simulink model "PID_Regler"  (R2019a)
settings: Solver=VariableStepAuto  StartTime=0.0  StopTime=10.0  RelTol=1e-3
values from neighbouring files (symbols this model uses):
  b = 0.1    [inv_pend.m]
  g = 9.8    [inv_pend.m]
  I = 0.006    [inv_pend.m]
  l = 0.3    [inv_pend.m]
  m = 0.5    [inv_pend.m]
  M = 0.5    [inv_pend.m]
libraries: simulink x1
settings Model: Creator=Naveen  LastModifiedBy=Naveen

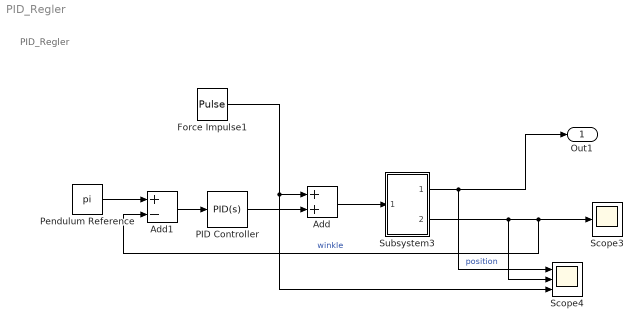
== system PID_Regler ==
  note: PID_Regler
  Add : Sum
  Add1 : Sum  Inputs=+-
  Force Impulse1 : DiscretePulseGenerator  PulseType=Time based  Amplitude=10  Period=100  PulseWidth=0.01  PhaseDelay=3
  PID Controller : simulink/Continuous/PID Controller  Controller=PID  Form=Parallel  TimeDomain=Continuous-time  SampleTime=-1  IntegratorMethod=Forward Euler  FilterMethod=Forward Euler  ControllerParametersSource=internal  P=100  I=1  D=20  UseFilter=on  N=100  TunerSelectOption=Transfer Function Based (PID Tuner App)  InitialConditionSource=internal  InitialConditionForIntegrator=0  InitialConditionForFilter=0  DifferentiatorICPrevScaledInput=0  ExternalReset=none  TrackingMode=off  Kt=1  LimitOutput=off  UpperSaturationLimit=inf  LowerSaturationLimit=-inf  LinearizeAsGain=on  AntiWindupMode=none  Kb=1  POutMin=[]  POutMax=[]  IOutMin=[]  IOutMax=[]  DOutMin=[]  DOutMax=[]  NOutMin=[]  NOutMax=[]  SumOutMin=[]  SumOutMax=[]  SaturationOutMin=[]  SaturationOutMax=[]  PParamMin=[]  PParamMax=[]  IParamMin=[]  IParamMax=[]  DParamMin=[]  DParamMax=[]  NParamMin=[]  NParamMax=[]  KbParamMin=[]  KbParamMax=[]  KtParamMin=[]  KtParamMax=[]  KbOutMin=[]  KbOutMax=[]  KtOutMin=[]  KtOutMax=[]  IntegratorOutMin=[]  IntegratorOutMax=[]  FilterOutMin=[]  FilterOutMax=[]  SumI1OutMin=[]  SumI1OutMax=[]  SumI2OutMin=[]  SumI2OutMax=[]  SumI3OutMin=[]  SumI3OutMax=[]  SumI4OutMin=[]  SumI4OutMax=[]  SumDOutMin=[]  SumDOutMax=[]  DifferentiatorOutMin=[]  DifferentiatorOutMax=[]  FilterDiffOutCoefMin=[]  FilterDiffOutCoefMax=[]  ReciprocalOutMin=[]  ReciprocalOutMax=[]  SumDenOutMin=[]  SumDenOutMax=[]  SumNumOutMin=[]  SumNumOutMax=[]  DivideOutMin=[]  DivideOutMax=[]  IntegratorContinuousStateAttributes=''  IntegratorStateMustResolveToSignalObject=off  IntegratorRTWStateStorageClass=Auto  FilterContinuousStateAttributes=''  FilterStateMustResolveToSignalObject=off  FilterRTWStateStorageClass=Auto  ParallelPVariant=InternalParameters  IdealPVariant=Disabled  IVariant=InternalParameters  DVariant=InternalParameters  IntegratorVariant=Continuous  SatVariant=Disabled  AWVariant=Passthrough  PCopyVariant=Disabled  TRVariant=Disabled  FdbkBlocksVariant=Forward  IdealPFdbkVariant=Disabled  SatFdbkVariant=Disabled  DerivativeFilterVariant=ContFilter  NVariant=InternalParameters  NCopyVariant=Disabled  FilterICVariant=InternalICsFilter  IntegratorICVariant=InternalICs  ExternalResetVariant=Disabled  TRSumVariant=Passthrough  SumFdbkVariant=Disabled  SumVariant=Sum_PID
  Pendulum Reference : Constant  Value=pi
  Scope3 : Scope
  Scope4 : Scope  NumInputPorts=3
  Subsystem3 : Subsystem
  Out1 : Outport
  wires:
  Pendulum Reference/1 -> Add1/1
  Force Impulse1/1 -> Scope4/3, Add/1
  Add1/1 -> PID Controller/1
  PID Controller/1 -> Add/2
  Add/1 -> Subsystem3/1(Force)
  Subsystem3/1(Position) -> Scope4/1, Out1/1  "position"
  Subsystem3/2(Angle) -> Scope4/2, Scope3/1, Add1/2  "winkle"

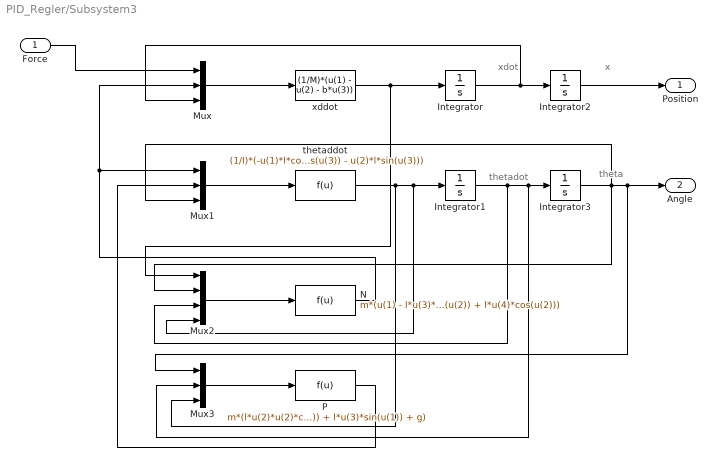
== system PID_Regler/Subsystem3 ==
  note: x
  note: thetadot
  note: theta
  note: xdot
  Force : Inport
  Integrator : Integrator  ContinuousStateAttributes='xdot'
  Integrator1 : Integrator  ContinuousStateAttributes='thetadot'
  Integrator2 : Integrator  ContinuousStateAttributes='x'
  Integrator3 : Integrator  InitialCondition=pi  ContinuousStateAttributes='theta'
  Mux : Mux  Inputs=3
  Mux1 : Mux  Inputs=3
  Mux2 : Mux
  Mux3 : Mux  Inputs=3
  N : Fcn  Expr=m*(u(1) - l*u(3)*u(3)*sin(u(2)) + l*u(4)*cos(u(2)))
  P : Fcn  Expr=m*(l*u(2)*u(2)*cos(u(1)) + l*u(3)*sin(u(1)) + g)
  thetaddot : Fcn  Expr=(1/I)*(-u(1)*l*cos(u(3)) - u(2)*l*sin(u(3)))
  xddot : Fcn  Expr=(1/M)*(u(1) - u(2) - b*u(3))
  Position : Outport
  Angle : Outport  Port=2
  wires:
  Integrator2/1 -> Position/1
  Integrator3/1 -> Mux2/2, Mux1/3, Angle/1, Mux3/1
  Mux3/1 -> P/1
  Force/1 -> Mux/1
  Integrator1/1 -> Mux2/3, Mux3/2, Integrator3/1
  xddot/1 -> Mux2/1, Integrator/1
  Integrator/1 -> Mux/3, Integrator2/1
  Mux1/1 -> thetaddot/1
  Mux2/1 -> N/1
  Mux/1 -> xddot/1
  N/1 -> Mux1/1, Mux/2
  thetaddot/1 -> Mux3/3, Mux2/4, Integrator1/1
  P/1 -> Mux1/2
